simulink model "motor_nucleo"  (R2020a)
settings: Solver=FixedStepDiscrete  StartTime=0.0  StopTime=10.0  RelTol=1e-3  EnableMultiTasking=on
libraries: TIMERS_Lib x3, GPIO_Lib x2, REG_Lib x2, simulink x1, STM32_Config_Lib x1, USART_Lib x1
settings Model: Creator=Gang  LastModifiedBy=tuziz
settings DataIOCC: LimitDataPoints=on  SaveFormat=Array  ReturnWorkspaceOutputs=off
settings OptimizationCC: DefaultParameterBehavior=Inlined  DefaultUnderspecifiedDataType=single  LifeSpan=1  EfficientTunableParamExpr=on
settings DebuggingCC: UnderspecifiedInitializationDetection=Classic  MergeDetectMultiDrivingBlocksExec=none  InheritedTsInSrcMsg=none  UniqueDataStoreMsg=error  AllowSymbolicDim=off  StrictBusMsg=ErrorOnBusTreatedAsVector  SFUnexpectedBacktrackingDiag=warning  SFNoUnconditionalDefaultTransitionDiag=warning  SFUndirectedBroadcastEventsDiag=error  SFExecutionAtInitializationDiag=none  ArithmeticOperatorsInVariantConditions=warning
settings HardwareCC: ProdBitPerPointer=32  ProdBitPerSizeT=32  ProdBitPerPtrDiffT=32  ProdLargestAtomicInteger=Integer  ProdWordSize=32  ProdHWDeviceType=STMicroelectronics->STM32 32-bit Cortex-M
settings ModelReferenceCC: PropagateSignalLabelsOutOfModel=off
settings SFSimCC: SimUseLocalCustomCode=off  CompileTimeRecursionLimit=0  EnableRuntimeRecursion=off  MATLABDynamicMemAlloc=off  CustomCodeUndefinedFunction=UseInterfaceOnly
settings RTWCC: Description=stm32 (Embedded Target)  SystemTargetFile=stm32.tlc  TemplateMakefile=stm32.tmf  GenerateReport=on  RTWUseLocalCustomCode=off
settings CodeAppCC: IgnoreCustomStorageClasses=off  CustomSymbolStrType=$N$R$M  SimulinkBlockComments=off
settings STFCustomTargetCC: TargetLangStandard=C99 (ISO)  ParMdlRefBuildCompliant=on  IncludeMdlTerminateFcn=off  CombineOutputUpdateFcns=on  ERTCustomFileBanners=on  SupportComplex=off  SupportContinuousTime=off  SupportNonInlinedSFcns=off  RemoveResetFunc=on  ParenthesesLevel=Maximum  CastingMode=Standards  MATLABClassNameForMDSCustomization=Simulink.SoftwareTarget.ERTCustomization  SystemTargetFile=stm32.tlc
settings ERTTargetCC: TargetLangStandard=C99 (ISO)  MultiwordLength=2048  CompOptLevelCompliant=off  ConcurrentExecutionCompliant=off  IncludeMdlTerminateFcn=off  SupportComplex=off  ParenthesesLevel=Maximum  CastingMode=Standards  ModelStepFunctionPrototypeControlCompliant=off  CPPClassGenCompliant=off  UseToolchainInfoCompliant=off  ERTSrcFileBannerTemplate=sourceFileTemplate.cgt  ERTHdrFileBannerTemplate=sourceFileTemplate.cgt  ERTDataSrcFileTemplate=sourceFileTemplate.cgt  ERTDataHdrFileTemplate=sourceFileTemplate.cgt  ERTCustomFileTemplate=customRoutineProcess.tlc  ConvertIfToSwitch=off  SuppressUnreachableDefaultCases=off  EnableSignedLeftShifts=off  EnableSignedRightShifts=off
settings ConfigComp: CovMetricSettings=dw  CovHtmlReporting=on  CovSaveCumulativeToWorkspaceVar=on  CovSaveSingleToWorkspaceVar=on  CovExternalEMLEnable=off  CovSFcnEnable=off

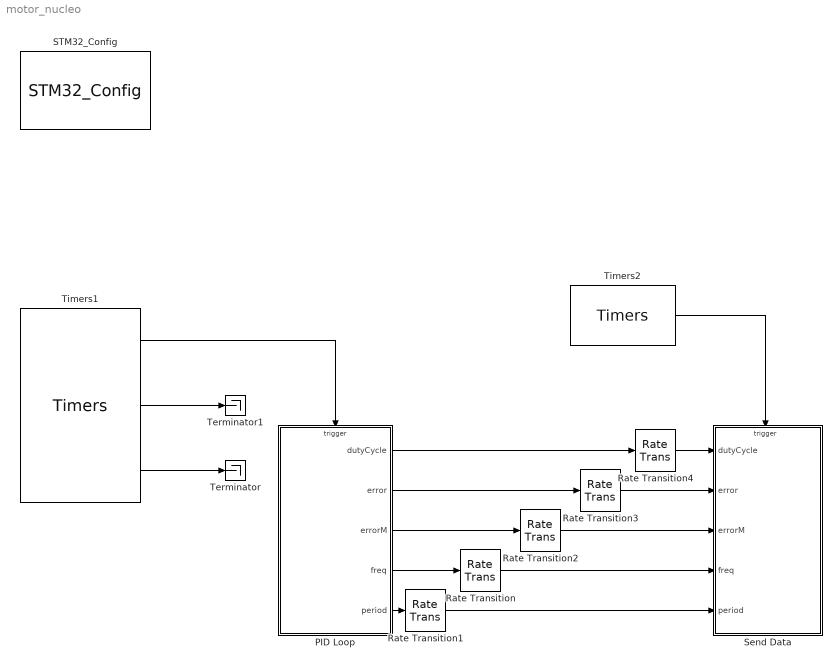
== system motor_nucleo ==
  PID Loop : Subsystem  TreatAsAtomicUnit=on
  Rate Transition{,1..4} (5 alike) : RateTransition  Deterministic=off
  STM32_Config : STM32_Config_Lib/STM32_Config  Priority=0  Project_Path=.\  Config_File=motor_nucleo.ioc  MCU_Name=STM32F412ZGTx
      settings: SourceProductName=Target Support Package - STM32 Adapter
  Send Data : Subsystem  TreatAsAtomicUnit=on
  Terminator : Terminator
  Terminator1 : Terminator
  Timers1 : TIMERS_Lib/Timers  currentTIM=TIM3  TIM_Name=TIM3  sysUsingTimer=off  TIM_APBClock=96000000  TIM_Set_Clk=off  TIM_Prescaler=96-1  TIM_Clock=1000000.00  Variable_frequency=off  TIM_Set_OutFreq=off  TIM_ARR=2000  Output_frequency=500.00  Repetition_counter=0  TIM_Mode=Up  TIM_DMA=none  TIM_IRQ=on  TIM_IRQ_ONLY=off  TIM_UP=on  TIM_TRG=off  TIM_COM=off  TIM_BRK=off  NbTIM=3  CH1_enable=on  CH1N_enable=off  CH1_type=Input_Capture  CH1_DMA=off  CH1_int=on  CH1_edge=Rising  CH1_div=1  CH1_variable_duty=off  CH1_set_pulse=off  CH1_output_duty=0.00  CH1_pulse=0  CH2_enable=off  CH2N_enable=off  CH2_type=Unknown  CH2_DMA=off  CH2_int=off  CH2_edge=Rising  CH2_div=1  CH2_variable_duty=off  CH2_set_pulse=off  CH2_output_duty=0.00  CH2_pulse=0  CH3_enable=off  CH3N_enable=off  CH3_type=Unknown  CH3_DMA=off  CH3_int=off  CH3_edge=Rising  CH3_div=1  CH3_variable_duty=off  CH3_set_pulse=off  CH3_output_duty=0.00  CH3_pulse=0  CH4_enable=off  CH4N_enable=off  CH4_type=Unknown  CH4_DMA=off  CH4_int=off  CH4_edge=Rising  CH4_div=1  CH4_variable_duty=off  CH4_set_pulse=off  CH4_output_duty=0.00  CH4_pulse=0
      settings: SourceProductName=Target Support Package - STM32 Adapter
  Timers2 : TIMERS_Lib/Timers  currentTIM=TIM7  TIM_Name=TIM7  sysUsingTimer=off  TIM_APBClock=96000000  TIM_Set_Clk=off  TIM_Prescaler=1920-1  TIM_Clock=50000.00  Variable_frequency=off  TIM_Set_OutFreq=off  TIM_ARR=500  Output_frequency=100.00  Repetition_counter=0  TIM_Mode=Up  TIM_DMA=none  TIM_IRQ=off  TIM_IRQ_ONLY=on  TIM_UP=on  TIM_TRG=off  TIM_COM=off  TIM_BRK=off  NbTIM=3  CH1_enable=off  CH1N_enable=off  CH1_type=Unknown  CH1_DMA=off  CH1_int=off  CH1_edge=Rising  CH1_div=1  CH1_variable_duty=off  CH1_set_pulse=off  CH1_output_duty=0.00  CH1_pulse=0  CH2_enable=off  CH2N_enable=off  CH2_type=Unknown  CH2_DMA=off  CH2_int=off  CH2_edge=Rising  CH2_div=1  CH2_variable_duty=off  CH2_set_pulse=off  CH2_output_duty=0.00  CH2_pulse=0  CH3_enable=off  CH3N_enable=off  CH3_type=Unknown  CH3_DMA=off  CH3_int=off  CH3_edge=Rising  CH3_div=1  CH3_variable_duty=off  CH3_set_pulse=off  CH3_output_duty=0.00  CH3_pulse=0  CH4_enable=off  CH4N_enable=off  CH4_type=Unknown  CH4_DMA=off  CH4_int=off  CH4_edge=Rising  CH4_div=1  CH4_variable_duty=off  CH4_set_pulse=off  CH4_output_duty=0.00  CH4_pulse=0
      settings: SourceProductName=Target Support Package - STM32 Adapter
  wires:
  Timers2/1 -> Send Data/Trigger
  Timers1/3 -> Terminator/1
  Timers1/2 -> Terminator1/1
  Timers1/1 -> PID Loop/Trigger
  PID Loop/4(freq) -> Rate Transition/1
  PID Loop/5(period) -> Rate Transition1/1
  Rate Transition/1 -> Send Data/4(freq)
  Rate Transition1/1 -> Send Data/5(period)
  Rate Transition2/1 -> Send Data/3(errorM)
  PID Loop/3(errorM) -> Rate Transition2/1
  PID Loop/2(error) -> Rate Transition3/1
  Rate Transition3/1 -> Send Data/2(error)
  Rate Transition4/1 -> Send Data/1(dutyCycle)
  PID Loop/1(dutyCycle) -> Rate Transition4/1

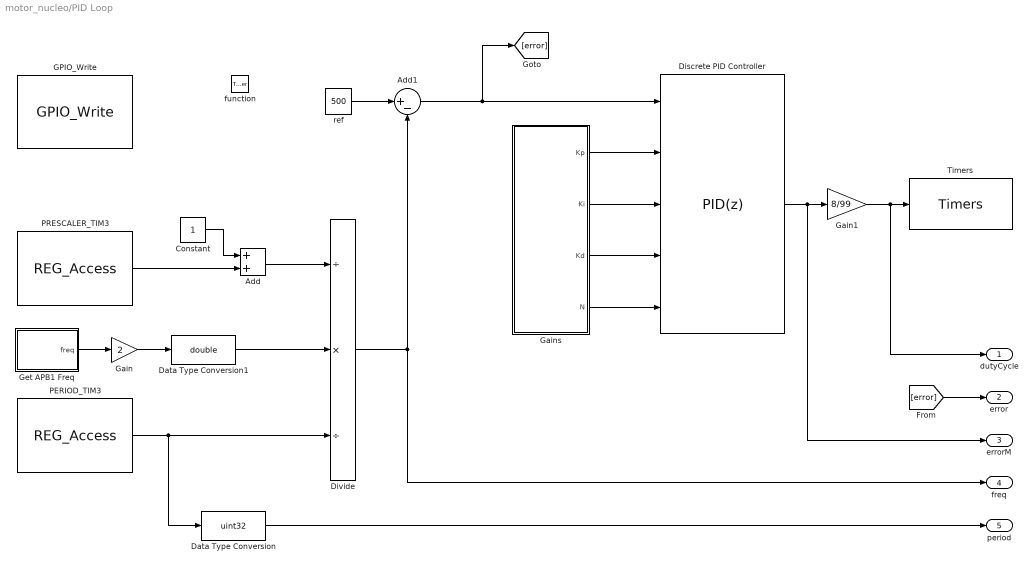
== system motor_nucleo/PID Loop ==
  function : TriggerPort  TriggerType=function-call  VariantControl=Variant
  Add : Sum  OutDataTypeStr=double
  Add1 : Sum  Inputs=|+-  OutDataTypeStr=double
  Constant : Constant  OutDataTypeStr=double
  Data Type Conversion : DataTypeConversion  OutDataTypeStr=uint32
  Data Type Conversion1 : DataTypeConversion  OutDataTypeStr=double
  Discrete PID Controller : simulink/Continuous/PID Controller  Controller=PID  Form=Parallel  TimeDomain=Discrete-time  UseExternalTs=off  SampleTime=-1  IntegratorMethod=Forward Euler  FilterMethod=Forward Euler  ControllerParametersSource=external  P=50.0  I=5  D=.5  UseFilter=on  N=100  TunerSelectOption=Transfer Function Based (PID Tuner App)  InitialConditionSource=internal  InitialConditionForIntegrator=0  InitialConditionForFilter=0  DifferentiatorICPrevScaledInput=0  ExternalReset=none  TrackingMode=off  Kt=1  LimitOutput=on  UpperSaturationLimit=1000  LowerSaturationLimit=0  LinearizeAsGain=off  AntiWindupMode=clamping  Kb=1  POutMin=[]  POutMax=[]  IOutMin=[]  IOutMax=[]  DOutMin=[]  DOutMax=[]  NOutMin=[]  NOutMax=[]  SumOutMin=[]  SumOutMax=[]  SaturationOutMin=[]  SaturationOutMax=[]  PParamMin=[]  PParamMax=[]  IParamMin=[]  IParamMax=[]  DParamMin=[]  DParamMax=[]  NParamMin=[]  NParamMax=[]  KbParamMin=[]  KbParamMax=[]  KtParamMin=[]  KtParamMax=[]  KbOutMin=[]  KbOutMax=[]  KtOutMin=[]  KtOutMax=[]  IntegratorOutMin=[]  IntegratorOutMax=[]  FilterOutMin=[]  FilterOutMax=[]  SumI1OutMin=[]  SumI1OutMax=[]  SumI2OutMin=[]  SumI2OutMax=[]  SumI3OutMin=[]  SumI3OutMax=[]  SumI4OutMin=[]  SumI4OutMax=[]  SumDOutMin=[]  SumDOutMax=[]  DifferentiatorOutMin=[]  DifferentiatorOutMax=[]  FilterDiffOutCoefMin=[]  FilterDiffOutCoefMax=[]  ReciprocalOutMin=[]  ReciprocalOutMax=[]  SumDenOutMin=[]  SumDenOutMax=[]  SumNumOutMin=[]  SumNumOutMax=[]  DivideOutMin=[]  DivideOutMax=[]  UdiffTsProdOutMin=[]  UdiffTsProdOutMax=[]  NTsProdOutMin=[]  NTsProdOutMax=[]  UintegralTsProdOutMin=[]  UintegralTsProdOutMax=[]  UngainTsProdOutMin=[]  UngainTsProdOutMax=[]  IntegratorContinuousStateAttributes=''  IntegratorStateMustResolveToSignalObject=off  IntegratorRTWStateStorageClass=Auto  FilterContinuousStateAttributes=''  FilterStateMustResolveToSignalObject=off  FilterRTWStateStorageClass=Auto  ParallelPVariant=ExternalParameters  IdealPVariant=Disabled  IVariant=ExternalParameters  DVariant=ExternalParameters  IntegratorVariant=Discrete  SatVariant=Enabled  AWVariant=DiscClampingParallel  PCopyVariant=Disabled  TRVariant=Disabled  FdbkBlocksVariant=Forward  IdealPFdbkVariant=Disabled  SatFdbkVariant=Disabled  DerivativeFilterVariant=ForwardEulerFilter  NVariant=ExternalParameters  NCopyVariant=Disabled  FilterICVariant=InternalICsFilter  IntegratorICVariant=InternalICs  ExternalResetVariant=Disabled  TRSumVariant=Passthrough  SumFdbkVariant=Disabled  SumVariant=Sum_PID  TsampFilterVariant=InternalTs  TsampNgainVariant=Passthrough  TsampIntegralVariant=Passthrough
  Divide : Product  Inputs=/*/  OutDataTypeStr=double
  GPIO_Write : GPIO_Lib/GPIO_Write  Port_name=GPIOB  Pin0=off  Toggle_Pin0=off  Pin1=off  Toggle_Pin1=off  Pin2=off  Toggle_Pin2=off  Pin3=off  Toggle_Pin3=off  Pin4=off  Toggle_Pin4=off  Pin5=off  Toggle_Pin5=off  Pin6=off  Toggle_Pin6=off  Pin7=on  Toggle_Pin7=on  Pin8=off  Toggle_Pin8=off  Pin9=off  Toggle_Pin9=off  Pin10=off  Toggle_Pin10=off  Pin11=off  Toggle_Pin11=off  Pin12=off  Toggle_Pin12=off  Pin13=off  Toggle_Pin13=off  Pin14=off  Toggle_Pin14=off  Pin15=off  Toggle_Pin15=off  PinList="GPIOB0  7GPIOG6"
      settings: SourceProductName=Target Support Package - STM32 Adapter
  Gain : Gain  Gain=2  ParamDataTypeStr=double  OutDataTypeStr=double
  Gain1 : Gain  Gain=8/99  OutDataTypeStr=double
  Gains : MATLAB Function  TreatAsAtomicUnit=on
  Get APB1 Freq : MATLAB Function  TreatAsAtomicUnit=on
  PERIOD_TIM3 : REG_Lib/REG_Access  Peripheral=TIM3  RegName=CCR1  RegRead=on  RegWrite=off  RegValueIn=off  RegEqual=on  RegAnd=off  RegOr=off  RegComplement=off  currentPeriph=TIM3
      settings: SourceProductName=Target Support Package - STM32 Adapter
  PRESCALER_TIM3 : REG_Lib/REG_Access  Peripheral=TIM3  RegName=PSC  RegRead=on  RegWrite=off  RegValueIn=off  RegEqual=on  RegAnd=off  RegOr=off  RegComplement=off  currentPeriph=TIM3
      settings: SourceProductName=Target Support Package - STM32 Adapter
  Timers : TIMERS_Lib/Timers  currentTIM=TIM12  TIM_Name=TIM12  sysUsingTimer=off  TIM_APBClock=96000000  TIM_Set_Clk=off  TIM_Prescaler=1920-1  TIM_Clock=50000.00  Variable_frequency=off  TIM_Set_OutFreq=off  TIM_ARR=100  Output_frequency=500.00  Repetition_counter=0  TIM_Mode=Up  TIM_DMA=none  TIM_IRQ=off  TIM_IRQ_ONLY=off  TIM_UP=off  TIM_TRG=off  TIM_COM=off  TIM_BRK=off  NbTIM=3  CH1_enable=on  CH1N_enable=off  CH1_type=Output_PWM  CH1_DMA=off  CH1_int=off  CH1_edge=Rising  CH1_div=1  CH1_variable_duty=on  CH1_set_pulse=off  CH1_output_duty=0.00  CH1_pulse=0  CH2_enable=off  CH2N_enable=off  CH2_type=Unknown  CH2_DMA=off  CH2_int=off  CH2_edge=Rising  CH2_div=1  CH2_variable_duty=off  CH2_set_pulse=off  CH2_output_duty=0.00  CH2_pulse=0  CH3_enable=off  CH3N_enable=off  CH3_type=Unknown  CH3_DMA=off  CH3_int=off  CH3_edge=Rising  CH3_div=1  CH3_variable_duty=off  CH3_set_pulse=off  CH3_output_duty=0.00  CH3_pulse=0  CH4_enable=off  CH4N_enable=off  CH4_type=Unknown  CH4_DMA=off  CH4_int=off  CH4_edge=Rising  CH4_div=1  CH4_variable_duty=off  CH4_set_pulse=off  CH4_output_duty=0.00  CH4_pulse=0
      settings: SourceProductName=Target Support Package - STM32 Adapter
  ref : Constant  Value=500  OutDataTypeStr=double
  dutyCycle : Outport
  error : Outport  Port=2
  errorM : Outport  Port=3
  freq : Outport  Port=4
  period : Outport  Port=5
  wires:
  Add/1 -> Divide/1
  Gain/1 -> Data Type Conversion1/1
  Data Type Conversion1/1 -> Divide/2
  Data Type Conversion/1 -> period/1
  PRESCALER_TIM3/1 -> Add/2
  Constant/1 -> Add/1
  PERIOD_TIM3/1 -> Data Type Conversion/1, Divide/3
  Get APB1 Freq/1(freq) -> Gain/1
  ref/1 -> Add1/1
  Divide/1 -> Add1/2, freq/1
  Add1/1 -> [error], Discrete PID Controller/1
  Gain1/1 -> Timers/1, dutyCycle/1
  Discrete PID Controller/1 -> Gain1/1, errorM/1
  [error] -> error/1
  Gains/1(Kp) -> Discrete PID Controller/2
  Gains/2(Ki) -> Discrete PID Controller/3
  Gains/3(Kd) -> Discrete PID Controller/4
  Gains/4(N) -> Discrete PID Controller/5

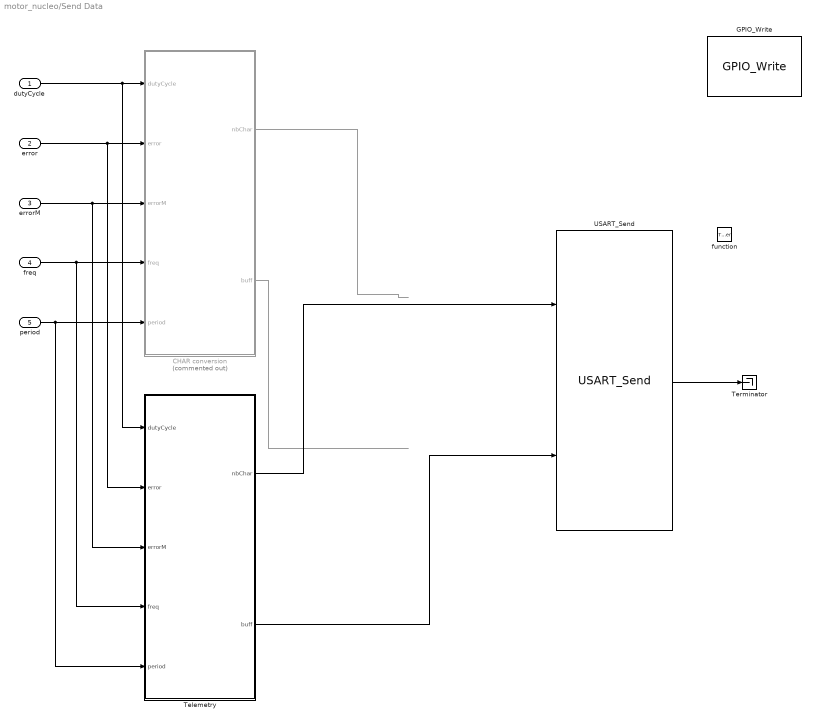
== system motor_nucleo/Send Data ==
  dutyCycle : Inport
  error : Inport  Port=2
  errorM : Inport  Port=3
  freq : Inport  Port=4
  period : Inport  Port=5
  function : TriggerPort  TriggerType=function-call  VariantControl=Variant
  CHAR conversion : MATLAB Function  Commented=on  TreatAsAtomicUnit=on
  GPIO_Write : GPIO_Lib/GPIO_Write  Port_name=GPIOB  Pin0=on  Toggle_Pin0=on  Pin1=off  Toggle_Pin1=off  Pin2=off  Toggle_Pin2=off  Pin3=off  Toggle_Pin3=off  Pin4=off  Toggle_Pin4=off  Pin5=off  Toggle_Pin5=off  Pin6=off  Toggle_Pin6=off  Pin7=off  Toggle_Pin7=off  Pin8=off  Toggle_Pin8=off  Pin9=off  Toggle_Pin9=off  Pin10=off  Toggle_Pin10=off  Pin11=off  Toggle_Pin11=off  Pin12=off  Toggle_Pin12=off  Pin13=off  Toggle_Pin13=off  Pin14=off  Toggle_Pin14=off  Pin15=off  Toggle_Pin15=off  PinList="GPIOB0  7GPIOG6"
      settings: SourceProductName=Target Support Package - STM32 Adapter
  Telemetry : MATLAB Function  TreatAsAtomicUnit=on
  Terminator : Terminator
  USART_Send : USART_Lib/USART_Send  USART_name=USART3  Buff_size=512  nbUsart=1  usartMode=Asynchronous  usartDma_Rx=off  usartDma_Tx=off  usartIt=off
      settings: SourceProductName=Target Support Package - STM32 Adapter
  wires:
  USART_Send/1 -> Terminator/1
  period/1 -> Telemetry/5(period), CHAR conversion/5(period)
  freq/1 -> Telemetry/4(freq), CHAR conversion/4(freq)
  dutyCycle/1 -> Telemetry/1(dutyCycle), CHAR conversion/1(dutyCycle)
  error/1 -> Telemetry/2(error), CHAR conversion/2(error)
  errorM/1 -> Telemetry/3(errorM), CHAR conversion/3(errorM)
  CHAR conversion/1(nbChar) -> ?
  CHAR conversion/2(buff) -> ?
  Telemetry/1(nbChar) -> USART_Send/1
  Telemetry/2(buff) -> USART_Send/2

== matlab function motor_nucleo/PID Loop/Get APB1 Freq ==
  data: freq output
function freq = fcn()
if coder.target('Sfun')
    % Executing in MATLAB, Buff is null
    freq = double(0);
else
    coder.cinclude('stm32f4xx_hal_rcc.h');
    
    % Executing in the generated code.
    freq = coder.ceval('HAL_RCC_GetPCLK1Freq');
end
end

== matlab function motor_nucleo/Send Data/CHAR conversion ==
  data: dutyCycle input; error input; errorM input; freq input; nbChar output uint16 size=1; buff output uint32 size=1; period input
function [nbChar, buff] = convert(dutyCycle,error,errorM,freq,period)
if coder.target('Sfun')
    % Executing in MATLAB, Buff is null
    buff = uint32(0);
    nbChar = uint16(0);
else
    coder.cinclude('stdio.h');
    coder.cinclude('main.h');
    coder.cinclude('getBuffPtr.h');

    % Executing in the generated code.
    string = char(zeros(1,90));
    stringSize = uint16(size(string,2));
    stringFormat = char([27,'[2J',27,'[H','Val: %u',13,10,'Error: %5.2f',13,10,'Scaled Error: %5.2f',13,10,'Freq: %5.2f',13,10,'dutyCycle: %5.2f',13,10,0]);
    coder.ceval('snprintf',coder.wref(string),stringSize,coder.rref(stringFormat),period,error,errorM,freq,dutyCycle);
    buff = coder.ceval('getBuffPtr',coder.rref(string));
    nbChar = stringSize;
end
end

== matlab function motor_nucleo/Send Data/Telemetry ==
  data: dutyCycle input; error input; errorM input; freq input; nbChar output uint16 size=1; buff output uint32 size=1; period input
function [nbChar, buff] = convert(dutyCycle,error,errorM,freq,period)
if coder.target('Sfun')
    % Executing in MATLAB, Buff is null
    buff = uint32(0);
    nbChar = uint16(0);
else
    coder.cinclude('stdio.h');
    coder.cinclude('main.h');
    coder.cinclude('getBuffPtr.h');

    % Executing in the generated code.
    string = char(zeros(1,50));
    stringSize = uint16(size(string,2));
    stringFormat = char(['%u,','%5.2f,','%5.2f,','%5.2f,','%5.2f',13,10,0]);
    coder.ceval('snprintf',coder.wref(string),stringSize,coder.rref(stringFormat),period,error,errorM,freq,dutyCycle);
    buff = coder.ceval('getBuffPtr',coder.rref(string));
    nbChar = stringSize - 4;
end
end

== matlab function motor_nucleo/PID Loop/Gains ==
  data: Kp output; Ki output; Kd output; N output
function [Kp,Ki,Kd,N] = fcn()
Kp = 2.0;
Ki = 0.8;
Kd = 30.0;
N = 100.0;
end
